simulink library "Pathfinding_lib"  (R2023b)
settings: Solver=VariableStepAuto  StartTime=0.0  StopTime=10.0  RelTol=1e-3
undefined symbols (not defined in the file): Spline_Max_Num_RefPoses, Spline_Num_Samples, Spline_Samples_Per_Pass, Spline_Tension, Spline_Velocity_Adjustment_Magnitude
libraries: $bdroot x39, simulink x4, matrix_library x1
settings Model: Creator=FIRSTMentor  LastModifiedBy=FIRSTMentor

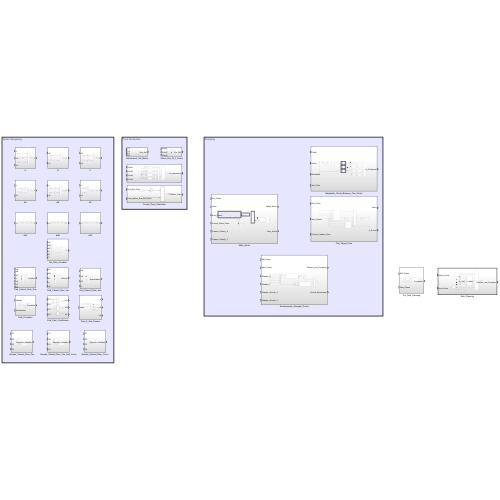
[thumbnail: Simulink's stored preview of the top-level diagram]
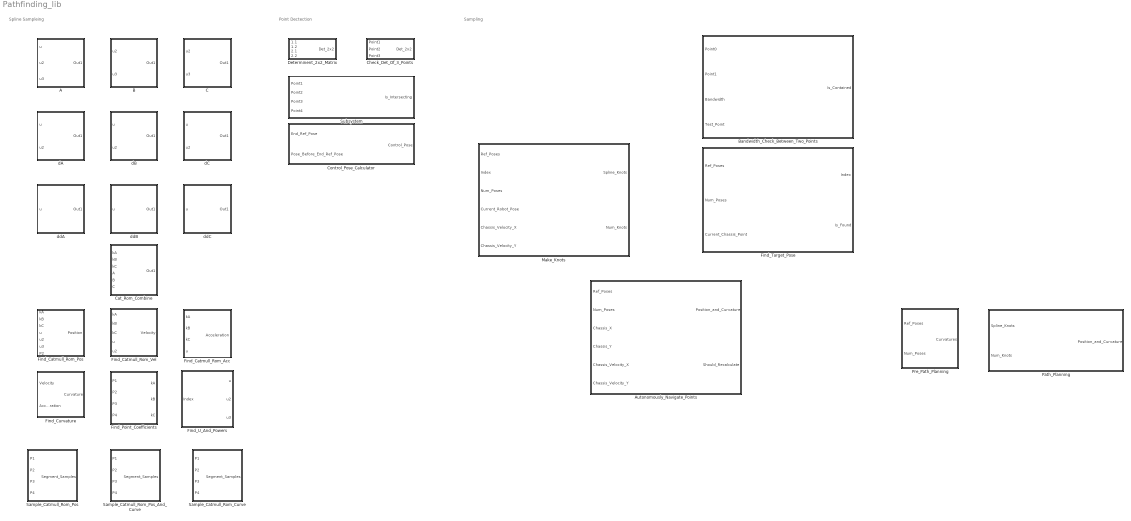
== system Pathfinding_lib ==
  note: Sampling
  note: Point Dectection
  note: Spline Sampleing
  A : Subsystem
  Autonomously_Navigate_Points : Subsystem
  B : Subsystem
  Bandwidth_Check_Between_Two_Points : Subsystem
  C : Subsystem
  Cat_Rom_Combine : Subsystem
  Check_Det_Of_3_Points : Subsystem
  Control_Pose_Calculator : Subsystem
  Determinent_2x2_Matrix : Subsystem
  Find_Catmull_Rom_Acc : Subsystem
  Find_Catmull_Rom_Pos : Subsystem
  Find_Catmull_Rom_Vel : Subsystem
  Find_Curvature : Subsystem
  Find_Point_Coefficients : Subsystem
  Find_Target_Pose : Subsystem
  Find_U_And_Powers : Subsystem
  Make_Knots : Subsystem
  Path_Planning : Subsystem  TreatAsAtomicUnit=on
  Pre_Path_Planning : Subsystem
  Sample_Catmull_Rom_Curve : Subsystem
  Sample_Catmull_Rom_Pos : Subsystem
  Sample_Catmull_Rom_Pos_And_Curve : Subsystem
  Subsystem : Subsystem
  dA : Subsystem
  dB : Subsystem
  dC : Subsystem
  ddA : Subsystem
  ddB : Subsystem
  ddC : Subsystem

== system Pathfinding_lib/A ==
  u : Inport
  u2 : Inport  Port=2
  u3 : Inport  Port=3
  Add : Sum  Inputs=+-+
  Gain : Gain  Gain=2
  Out1 : Outport
  wires:
  Add/1 -> Out1/1
  u/1 -> Add/1
  u2/1 -> Gain/1
  Gain/1 -> Add/2
  u3/1 -> Add/3

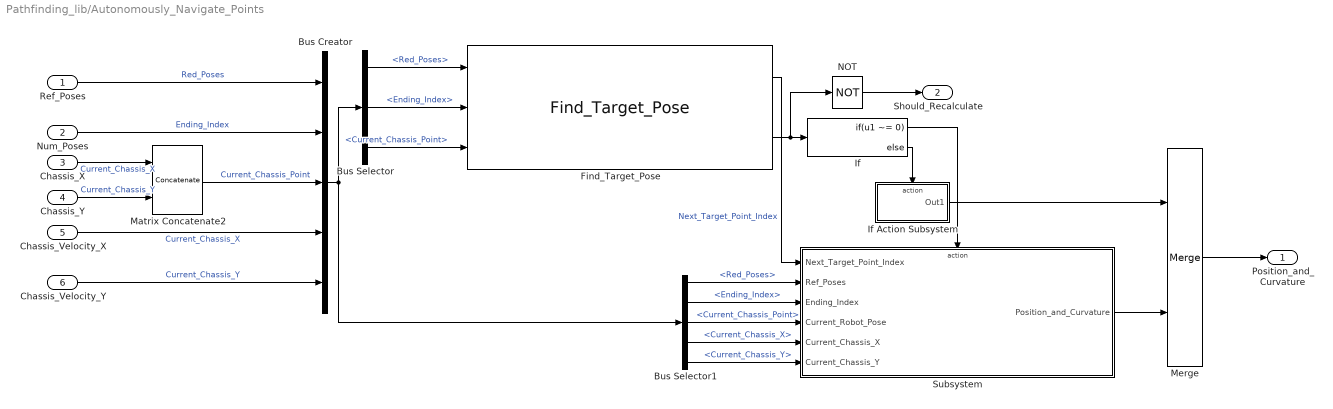
== system Pathfinding_lib/Autonomously_Navigate_Points ==
  Ref_Poses : Inport  OutDataTypeStr=double  PortDimensions=[Spline_Max_Num_RefPoses 2]
  Num_Poses : Inport  Port=2  OutDataTypeStr=int32  Unit=1  PortDimensions=1
  Chassis_X : Inport  Port=3  OutDataTypeStr=double  Unit=m  PortDimensions=1
  Chassis_Y : Inport  Port=4  OutDataTypeStr=double  Unit=m  PortDimensions=1
  Chassis_Velocity_X : Inport  Port=5  OutDataTypeStr=double  Unit=m  PortDimensions=1
  Chassis_Velocity_Y : Inport  Port=6  OutDataTypeStr=double  Unit=m  PortDimensions=1
  Bus Creator : BusCreator  Inputs=5
  Bus Selector : BusSelector  OutputSignals=Red_Poses,Ending_Index,Current_Chassis_Point
  Bus Selector1 : BusSelector  OutputSignals=Red_Poses,Ending_Index,Current_Chassis_Point,Current_Chassis_X,Current_Chassis_Y
  Find_Target_Pose : $bdroot/Find_Target_Pose  SystemSampleTime=-1  VariantActivationTime=update diagram  AllowFlexibleInterface=on  Latency=0  AutoFrameSizeCalculation=off
  If : If  IfExpression=u1 ~= 0
  If Action Subsystem : Subsystem  TreatAsAtomicUnit=on
  Matrix Concatenate2 : Concatenate  Mode=Multidimensional array  ConcatenateDimension=2
  Merge : Merge
  NOT : Logic  Operator=NOT  IconShape=distinctive  AllPortsSameDT=off  OutDataTypeStr=boolean
  Subsystem : Subsystem
  Position_and_Curvature : Outport  PortDimensions=[Spline_Num_Samples,3,2]
  Should_Recalculate : Outport  Port=2
  wires:
  Chassis_X/1 -> Matrix Concatenate2/1  "Current_Chassis_X"
  Chassis_Y/1 -> Matrix Concatenate2/2  "Current_Chassis_Y"
  Ref_Poses/1 -> Bus Creator/1  "Red_Poses"
  Matrix Concatenate2/1 -> Bus Creator/3  "Current_Chassis_Point"
  Num_Poses/1 -> Bus Creator/2  "Ending_Index"
  Find_Target_Pose/2 -> NOT/1, If/1
  Find_Target_Pose/1 -> Subsystem/1(Next_Target_Point_Index)  "Next_Target_Point_Index"
  Chassis_Velocity_X/1 -> Bus Creator/4  "Current_Chassis_X"
  Chassis_Velocity_Y/1 -> Bus Creator/5  "Current_Chassis_Y"
  Subsystem/1(Position_and_Curvature) -> Merge/2
  If/1 -> Subsystem/Action
  Bus Creator/1 -> Bus Selector1/1, Bus Selector/1
  Bus Selector/1 -> Find_Target_Pose/1  "<Red_Poses>"
  Bus Selector/2 -> Find_Target_Pose/2  "<Ending_Index>"
  Bus Selector/3 -> Find_Target_Pose/3  "<Current_Chassis_Point>"
  Bus Selector1/1 -> Subsystem/2(Ref_Poses)  "<Red_Poses>"
  Bus Selector1/2 -> Subsystem/3(Ending_Index)  "<Ending_Index>"
  Bus Selector1/3 -> Subsystem/4(Current_Robot_Pose)  "<Current_Chassis_Point>"
  Bus Selector1/4 -> Subsystem/5(Current_Chassis_X)  "<Current_Chassis_X>"
  Bus Selector1/5 -> Subsystem/6(Current_Chassis_Y)  "<Current_Chassis_Y>"
  NOT/1 -> Should_Recalculate/1
  If/2 -> If Action Subsystem/Action
  If Action Subsystem/1(Out1) -> Merge/1
  Merge/1 -> Position_and_Curvature/1

== system Pathfinding_lib/B ==
  u2 : Inport
  u3 : Inport  Port=2
  Add : Sum  Inputs=+-
  Out1 : Outport
  wires:
  Add/1 -> Out1/1
  u3/1 -> Add/2
  u2/1 -> Add/1

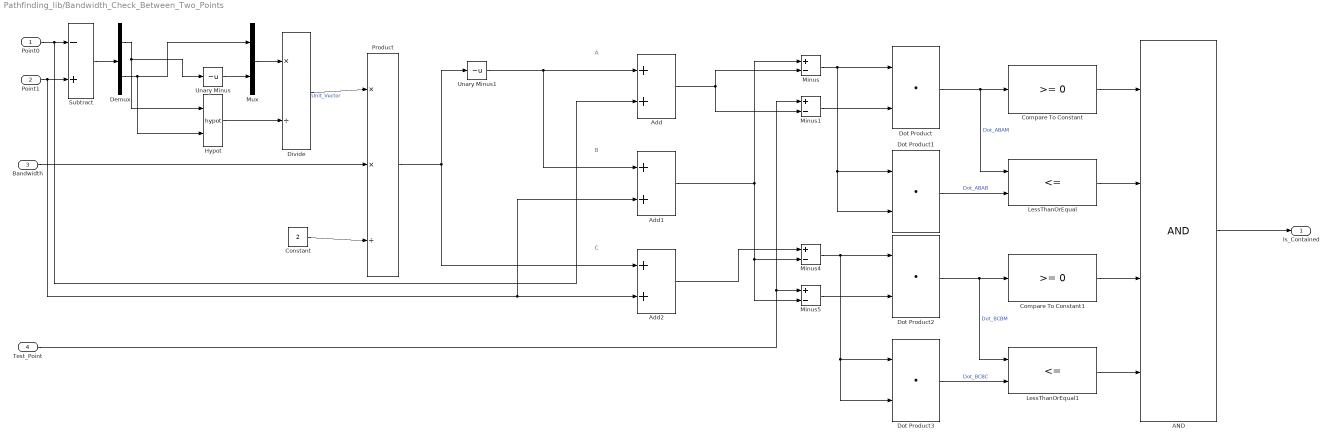
== system Pathfinding_lib/Bandwidth_Check_Between_Two_Points ==
  note: A
  note: B
  note: C
  Point0 : Inport  Unit=m  PortDimensions=[1 2]
  Point1 : Inport  Port=2  Unit=m  PortDimensions=[1 2]
  Bandwidth : Inport  Port=3  PortDimensions=1
  Test_Point : Inport  Port=4  Unit=m  PortDimensions=[1 2]
  AND : Logic  Inputs=4  IconShape=distinctive  AllPortsSameDT=off  OutDataTypeStr=boolean
  Add : Sum
  Add1 : Sum
  Add2 : Sum
  Compare To Constant : simulink/Logic and Bit Operations/Compare To Constant  relop=>=  const=0  OutDataTypeStr=boolean
  Compare To Constant1 : simulink/Logic and Bit Operations/Compare To Constant  relop=>=  const=0  OutDataTypeStr=boolean
  Constant : Constant  Value=2
  Demux : Demux  Outputs=2
  Divide : Product  Inputs=*/
  Dot Product{,1..3} (4 alike) : DotProduct  OutDataTypeStr=Inherit: Inherit via internal rule
  Hypot : Math  Operator=hypot
  LessThanOrEqual : RelationalOperator  Operator=<=  OutDataTypeStr=boolean  RndMeth=Simplest  InputSameDT=off
  LessThanOrEqual1 : RelationalOperator  Operator=<=  OutDataTypeStr=boolean  RndMeth=Simplest  InputSameDT=off
  Minus{,1,4..5} (4 alike) : Sum  Inputs=+-
  Mux : Mux  Inputs=2
  Product : Product  Inputs=**/
  Subtract : Sum  Inputs=-+
  Unary Minus : UnaryMinus
  Unary Minus1 : UnaryMinus
  Is_Contained : Outport
  wires:
  Point0/1 -> Add/2, Subtract/1
  Point1/1 -> Subtract/2, Add1/2, Add2/2
  Subtract/1 -> Demux/1
  Demux/2 -> Hypot/2, Mux/1
  Unary Minus/1 -> Mux/2
  Demux/1 -> Hypot/1, Unary Minus/1
  Mux/1 -> Divide/1
  Hypot/1 -> Divide/2
  Divide/1 -> Product/1  "Unit_Vector"
  Bandwidth/1 -> Product/2
  Constant/1 -> Product/3
  Product/1 -> Add2/1, Unary Minus1/1
  Unary Minus1/1 -> Add1/1, Add/1
  Minus1/1 -> Dot Product/2
  Dot Product/1 -> LessThanOrEqual/1, Compare To Constant/1  "Dot_ABAM"
  Dot Product1/1 -> LessThanOrEqual/2  "Dot_ABAB"
  Minus/1 -> Dot Product1/2, Dot Product1/1, Dot Product/1
  Dot Product2/1 -> Compare To Constant1/1, LessThanOrEqual1/1  "Dot_BCBM"
  Minus5/1 -> Dot Product2/2
  Dot Product3/1 -> LessThanOrEqual1/2  "Dot_BCBC"
  Minus4/1 -> Dot Product3/1, Dot Product3/2, Dot Product2/1
  Add1/1 -> Minus5/2, Minus4/2, Minus/1
  Add/1 -> Minus1/2, Minus/2
  Add2/1 -> Minus4/1
  Test_Point/1 -> Minus1/1, Minus5/1
  AND/1 -> Is_Contained/1
  Compare To Constant/1 -> AND/1
  Compare To Constant1/1 -> AND/3
  LessThanOrEqual/1 -> AND/2
  LessThanOrEqual1/1 -> AND/4

== system Pathfinding_lib/C ==
  u2 : Inport
  u3 : Inport  Port=2
  Add : Sum  Inputs=+-
  Gain : Gain  Gain=3
  Gain1 : Gain  Gain=2
  Out1 : Outport
  wires:
  u2/1 -> Gain/1
  u3/1 -> Gain1/1
  Gain/1 -> Add/1
  Gain1/1 -> Add/2
  Add/1 -> Out1/1

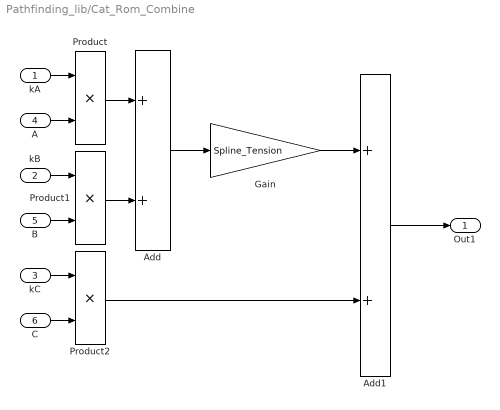
== system Pathfinding_lib/Cat_Rom_Combine ==
  kA : Inport
  kB : Inport  Port=2
  kC : Inport  Port=3
  A : Inport  Port=4
  B : Inport  Port=5
  C : Inport  Port=6
  Add : Sum  Inputs=2
  Add1 : Sum
  Gain : Gain  Gain=Spline_Tension
  Product : Product
  Product1 : Product
  Product2 : Product
  Out1 : Outport
  wires:
  kA/1 -> Product/1
  A/1 -> Product/2
  kC/1 -> Product2/1
  C/1 -> Product2/2
  kB/1 -> Product1/1
  B/1 -> Product1/2
  Product/1 -> Add/1
  Product1/1 -> Add/2
  Product2/1 -> Add1/2
  Add/1 -> Gain/1
  Add1/1 -> Out1/1
  Gain/1 -> Add1/1

== system Pathfinding_lib/Check_Det_Of_3_Points ==
  Point1 : Inport
  Point2 : Inport  Port=2
  Point3 : Inport  Port=3
  Demux : Demux  Outputs=2
  Demux1 : Demux  Outputs=2
  Demux2 : Demux  Outputs=2
  Determinent_2x2_Matrix : $bdroot/Determinent_2x2_Matrix  SystemSampleTime=-1  VariantActivationTime=update diagram  Latency=0  AutoFrameSizeCalculation=off
  Minus{,1..3} (4 alike) : Sum  Inputs=+-
  Det_2x2 : Outport
  wires:
  Determinent_2x2_Matrix/1 -> Det_2x2/1
  Minus/1 -> Determinent_2x2_Matrix/1
  Minus1/1 -> Determinent_2x2_Matrix/2
  Minus2/1 -> Determinent_2x2_Matrix/3
  Minus3/1 -> Determinent_2x2_Matrix/4
  Point1/1 -> Demux/1  "Point1"
  Point2/1 -> Demux1/1  "Point2"
  Point3/1 -> Demux2/1  "Point3"
  Demux/1 -> Minus/1  "Point1_X"
  Demux/2 -> Minus2/1  "Point1_Y"
  Demux1/1 -> Minus1/1  "Point2_X"
  Demux1/2 -> Minus3/1  "Point2_Y"
  Demux2/1 -> Minus2/2, Minus1/2, Minus/2  "Point3_X"
  Demux2/2 -> Minus3/2  "Point3_Y"

== system Pathfinding_lib/Control_Pose_Calculator ==
  End_Ref_Pose : Inport
  Pose_Before_End_Ref_Pose : Inport  Port=2
  Gain : Gain  Gain=2
  Subtract : Sum  Inputs=+-
  Control_Pose : Outport
  wires:
  End_Ref_Pose/1 -> Gain/1
  Gain/1 -> Subtract/1
  Pose_Before_End_Ref_Pose/1 -> Subtract/2
  Subtract/1 -> Control_Pose/1

== system Pathfinding_lib/Determinent_2x2_Matrix ==
  1.1 : Inport
  1.2 : Inport  Port=2
  2.1 : Inport  Port=3
  2.2 : Inport  Port=4
  Minus : Sum  Inputs=+-
  Product : Product
  Product1 : Product
  Det_2x2 : Outport
  wires:
  1.1/1 -> Product/1
  2.2/1 -> Product/2
  1.2/1 -> Product1/1
  2.1/1 -> Product1/2
  Product/1 -> Minus/1
  Product1/1 -> Minus/2
  Minus/1 -> Det_2x2/1

== system Pathfinding_lib/Find_Catmull_Rom_Acc ==
  kA : Inport  PortDimensions=[1 2]
  kB : Inport  Port=2  PortDimensions=[1 2]
  kC : Inport  Port=3  PortDimensions=[1 2]
  u : Inport  Port=4  PortDimensions=1
  Cat_Rom_Combine : $bdroot/Cat_Rom_Combine  SystemSampleTime=-1  VariantActivationTime=update diagram  AllowFlexibleInterface=on  Latency=0  AutoFrameSizeCalculation=off
  ddA : $bdroot/ddA  SystemSampleTime=-1  VariantActivationTime=update diagram  AllowFlexibleInterface=on  Latency=0  AutoFrameSizeCalculation=off
  ddB : $bdroot/ddB  SystemSampleTime=-1  VariantActivationTime=update diagram  AllowFlexibleInterface=on  Latency=0  AutoFrameSizeCalculation=off
  ddC : $bdroot/ddC  SystemSampleTime=-1  VariantActivationTime=update diagram  AllowFlexibleInterface=on  Latency=0  AutoFrameSizeCalculation=off
  Acceleration : Outport
  wires:
  kA/1 -> Cat_Rom_Combine/1
  kB/1 -> Cat_Rom_Combine/2
  kC/1 -> Cat_Rom_Combine/3
  ddA/1 -> Cat_Rom_Combine/4
  ddB/1 -> Cat_Rom_Combine/5
  ddC/1 -> Cat_Rom_Combine/6
  Cat_Rom_Combine/1 -> Acceleration/1
  u/1 -> ddA/1, ddC/1, ddB/1

== system Pathfinding_lib/Find_Catmull_Rom_Pos ==
  kA : Inport  PortDimensions=[1 2]
  kB : Inport  Port=2  PortDimensions=[1 2]
  kC : Inport  Port=3  PortDimensions=[1 2]
  u : Inport  Port=4  PortDimensions=1
  u2 : Inport  Port=5  PortDimensions=1
  u3 : Inport  Port=6  PortDimensions=1
  P2 : Inport  Port=7  PortDimensions=[1 2]
  A : $bdroot/A  SystemSampleTime=-1  VariantActivationTime=update diagram  AllowFlexibleInterface=on  Latency=0  AutoFrameSizeCalculation=off
  B : $bdroot/B  SystemSampleTime=-1  VariantActivationTime=update diagram  AllowFlexibleInterface=on  Latency=0  AutoFrameSizeCalculation=off
  C : $bdroot/C  SystemSampleTime=-1  VariantActivationTime=update diagram  AllowFlexibleInterface=on  Latency=0  AutoFrameSizeCalculation=off
  Cat_Rom_Combine : $bdroot/Cat_Rom_Combine  SystemSampleTime=-1  VariantActivationTime=update diagram  AllowFlexibleInterface=on  Latency=0  AutoFrameSizeCalculation=off
  Sum : Sum  Inputs=|++
  Position : Outport
  wires:
  u/1 -> A/1
  u2/1 -> C/1, B/1, A/2
  u3/1 -> C/2, B/2, A/3
  kA/1 -> Cat_Rom_Combine/1
  kB/1 -> Cat_Rom_Combine/2
  kC/1 -> Cat_Rom_Combine/3
  A/1 -> Cat_Rom_Combine/4
  B/1 -> Cat_Rom_Combine/5
  C/1 -> Cat_Rom_Combine/6
  P2/1 -> Sum/2
  Cat_Rom_Combine/1 -> Sum/1
  Sum/1 -> Position/1

== system Pathfinding_lib/Find_Catmull_Rom_Vel ==
  kA : Inport  PortDimensions=[1 2]
  kB : Inport  Port=2  PortDimensions=[1 2]
  kC : Inport  Port=3  PortDimensions=[1 2]
  u : Inport  Port=4  PortDimensions=1
  u2 : Inport  Port=5  PortDimensions=1
  Cat_Rom_Combine : $bdroot/Cat_Rom_Combine  SystemSampleTime=-1  VariantActivationTime=update diagram  AllowFlexibleInterface=on  Latency=0  AutoFrameSizeCalculation=off
  dA : $bdroot/dA  SystemSampleTime=-1  VariantActivationTime=update diagram  AllowFlexibleInterface=on  Latency=0  AutoFrameSizeCalculation=off
  dB : $bdroot/dB  SystemSampleTime=-1  VariantActivationTime=update diagram  AllowFlexibleInterface=on  Latency=0  AutoFrameSizeCalculation=off
  dC : $bdroot/dC  SystemSampleTime=-1  VariantActivationTime=update diagram  AllowFlexibleInterface=on  Latency=0  AutoFrameSizeCalculation=off
  Velocity : Outport
  wires:
  kA/1 -> Cat_Rom_Combine/1
  kB/1 -> Cat_Rom_Combine/2
  kC/1 -> Cat_Rom_Combine/3
  dA/1 -> Cat_Rom_Combine/4
  dB/1 -> Cat_Rom_Combine/5
  dC/1 -> Cat_Rom_Combine/6
  Cat_Rom_Combine/1 -> Velocity/1
  u/1 -> dC/1, dB/1, dA/1
  u2/1 -> dC/2, dB/2, dA/2

== system Pathfinding_lib/Find_Curvature ==
  Velocity : Inport  PortDimensions=[1 2]
  Acceleration : Inport  Port=2  PortDimensions=[1 2]
  Abs : Abs  SaturateOnIntegerOverflow=off
  Constant1 : Constant  Value=3
  Demux : Demux  Outputs=2
  Divide : Product  Inputs=*/
  Hypot : Math  Operator=hypot
  MATLAB Function : MATLAB Function  TreatAsAtomicUnit=on
  Matrix Concatenate : Concatenate  Mode=Multidimensional array
  Power1 : Math  Operator=pow
  Curvature : Outport  PortDimensions=1
  wires:
  Divide/1 -> Curvature/1
  Velocity/1 -> Demux/1, Matrix Concatenate/1
  Acceleration/1 -> Matrix Concatenate/2
  Matrix Concatenate/1 -> MATLAB Function/1(u)
  MATLAB Function/1(y) -> Abs/1
  Constant1/1 -> Power1/2
  Hypot/1 -> Power1/1
  Abs/1 -> Divide/1
  Power1/1 -> Divide/2
  Demux/1 -> Hypot/1
  Demux/2 -> Hypot/2

== system Pathfinding_lib/Find_Point_Coefficients ==
  P1 : Inport
  P2 : Inport  Port=2
  P3 : Inport  Port=3
  P4 : Inport  Port=4
  Minus : Sum  Inputs=+-
  Minus1 : Sum  Inputs=+-
  Minus2 : Sum  Inputs=+-
  kA : Outport
  kB : Outport  Port=2
  kC : Outport  Port=3
  wires:
  P2/1 -> Minus2/2, Minus1/1
  P1/1 -> Minus/2
  P3/1 -> Minus2/1, Minus/1
  P4/1 -> Minus1/2
  Minus/1 -> kA/1
  Minus1/1 -> kB/1
  Minus2/1 -> kC/1

== system Pathfinding_lib/Find_Target_Pose ==
  Ref_Poses : Inport  OutDataTypeStr=double  PortDimensions=[Spline_Max_Num_RefPoses 2]
  Num_Poses : Inport  Port=2  Unit=1  PortDimensions=1
  Current_Chassis_Point : Inport  Port=3  OutDataTypeStr=double  Unit=m  PortDimensions=[1 2]
  Bandwidth : Constant  Value=2
  Circle_Checks : Subsystem  TreatAsAtomicUnit=on
  Constant : Constant
  If : If  IfExpression=u1 == 0  ShowElse=off
  OR : Logic  Operator=OR  IconShape=distinctive  AllPortsSameDT=off  OutDataTypeStr=boolean
  Rectangle_Checks : Subsystem  TreatAsAtomicUnit=on
  Sum : Sum  Inputs=|++  OutDataTypeStr=int32
  Switch : Switch  Criteria=u2 ~= 0  SaturateOnIntegerOverflow=off  InputSameDT=off
  Index : Outport
  Is_Found : Outport  Port=2
  wires:
  Rectangle_Checks/2(Is_Found) -> Switch/2, OR/1, If/1
  Switch/1 -> Sum/1
  If/1 -> Circle_Checks/Action
  Num_Poses/1 -> Rectangle_Checks/2(Num_Poses), Circle_Checks/2(Num_Poses)  "Ending_Index"
  Current_Chassis_Point/1 -> Rectangle_Checks/3(Test_Point), Circle_Checks/3(Test_Point)  "Current_Chassis_Point"
  Ref_Poses/1 -> Rectangle_Checks/1(Ref_Poses), Circle_Checks/1(Ref_Poses)
  Rectangle_Checks/1(Index) -> Switch/1
  Circle_Checks/1(Index) -> Switch/3
  Bandwidth/1 -> Rectangle_Checks/4(Bandwidth), Circle_Checks/4(Bandwidth)
  Sum/1 -> Index/1  "Next_Target_Point_Index"
  OR/1 -> Is_Found/1
  Circle_Checks/2(Is_Found) -> OR/2
  Constant/1 -> Sum/2

== system Pathfinding_lib/Find_U_And_Powers ==
  Index : Inport
  Bias : Bias  Bias=-1  SaturateOnIntegerOverflow=off
  Constant : Constant  Value=2
  Constant1 : Constant  Value=3
  Constant2 : Constant  Value=Spline_Num_Samples-1
  Divide : Product  Inputs=*/
  Power : Math  Operator=pow
  Power1 : Math  Operator=pow
  u : Outport
  u2 : Outport  Port=2
  u3 : Outport  Port=3
  wires:
  Bias/1 -> Divide/1
  Constant2/1 -> Divide/2
  Power/1 -> u2/1  "u2"
  Power1/1 -> u3/1  "u3"
  Constant/1 -> Power/2
  Divide/1 -> u/1, Power1/1, Power/1  "u"
  Constant1/1 -> Power1/2
  Index/1 -> Bias/1

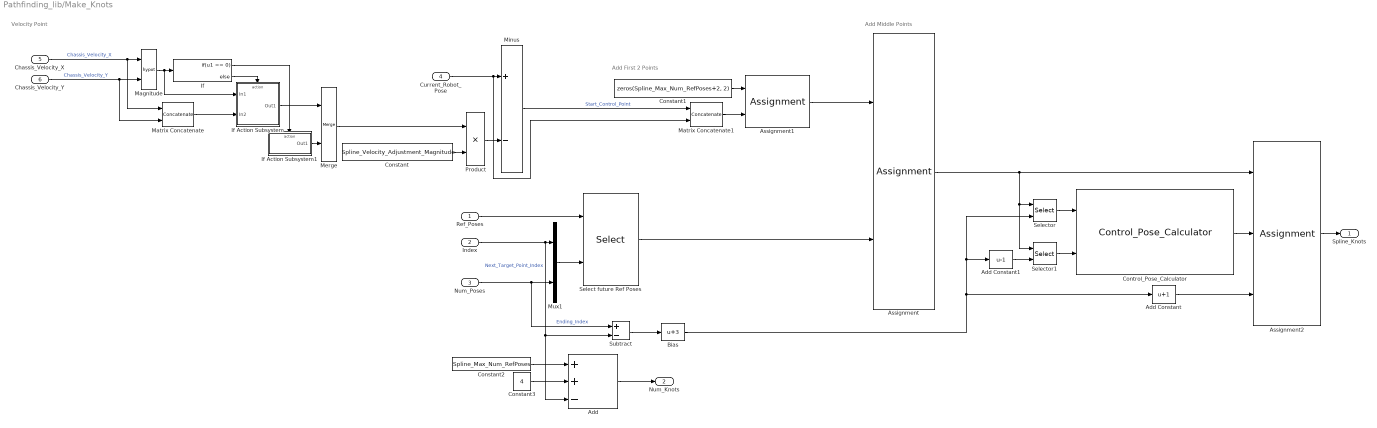
== system Pathfinding_lib/Make_Knots ==
  note: Add Middle Points
  note: Add First 2 Points
  note: Velocity Point
  Ref_Poses : Inport
  Index : Inport  Port=2
  Num_Poses : Inport  Port=3
  Current_Robot_Pose : Inport  Port=4
  Chassis_Velocity_X : Inport  Port=5
  Chassis_Velocity_Y : Inport  Port=6
  Add : Sum  Inputs=++-
  Add Constant : Bias  Bias=1  SaturateOnIntegerOverflow=off
  Add Constant1 : Bias  Bias=-1  SaturateOnIntegerOverflow=off
  Assignment : Assignment  NumberOfDimensions=2  DiagnosticForDimensions=Warning  IndexOptions=Starting index (dialog),Assign all  Indices=3,1  OutputSizes=1,1
  Assignment1 : Assignment  NumberOfDimensions=2  DiagnosticForDimensions=Warning  IndexOptions=Starting index (dialog),Assign all  Indices=1,1  OutputSizes=1,1
  Assignment2 : Assignment  NumberOfDimensions=2  DiagnosticForDimensions=Warning  IndexOptions=Index vector (port),Assign all  Indices=1,1  OutputSizes=1,1
  Bias : Bias  Bias=3  SaturateOnIntegerOverflow=off
  Constant : Constant  Value=Spline_Velocity_Adjustment_Magnitude
  Constant1 : Constant  Value=zeros(Spline_Max_Num_RefPoses+2, 2)
  Constant2 : Constant  Value=Spline_Max_Num_RefPoses
  Constant3 : Constant  Value=4
  Control_Pose_Calculator : $bdroot/Control_Pose_Calculator  SystemSampleTime=-1  VariantActivationTime=update diagram  AllowFlexibleInterface=on  Latency=0  AutoFrameSizeCalculation=off
  If : If  IfExpression=u1 == 0
  If Action Subsystem : Subsystem  TreatAsAtomicUnit=on
  If Action Subsystem1 : Subsystem  TreatAsAtomicUnit=on
  Magnitude : Math  Operator=hypot
  Matrix Concatenate : Concatenate  Mode=Multidimensional array  ConcatenateDimension=2
  Matrix Concatenate1 : Concatenate  Mode=Multidimensional array
  Merge : Merge
  Minus : Sum  Inputs=+-
  Mux1 : Mux  Inputs=2
  Product : Product
  Select future Ref Poses : Selector  NumberOfDimensions=2  InputPortWidth=3  IndexOptions=Starting and ending indices (port),Select all  Indices=[1 3],1  OutputSizes=1,1
  Selector : Selector  NumberOfDimensions=2  InputPortWidth=3  IndexOptions=Index vector (port),Select all  Indices=[1 3],1  OutputSizes=1,1
  Selector1 : Selector  NumberOfDimensions=2  InputPortWidth=3  IndexOptions=Index vector (port),Select all  Indices=[1 3],1  OutputSizes=1,1
  Subtract : Sum  Inputs=+-
  Spline_Knots : Outport
  Num_Knots : Outport  Port=2
  wires:
  Minus/1 -> Matrix Concatenate1/1  "Start_Control_Point"
  Matrix Concatenate1/1 -> Assignment1/2
  Selector/1 -> Control_Pose_Calculator/1
  Add Constant/1 -> Assignment2/3
  Product/1 -> Minus/2
  Current_Robot_Pose/1 -> Matrix Concatenate1/2, Minus/1
  Assignment/1 -> Assignment2/1, Selector/1, Selector1/1
  Index/1 -> Subtract/2, Add/3, Mux1/1  "Next_Target_Point_Index"
  Matrix Concatenate/1 -> If Action Subsystem/2(In2)
  Selector1/1 -> Control_Pose_Calculator/2
  Magnitude/1 -> If Action Subsystem/1(In1), If/1
  Assignment1/1 -> Assignment/1
  Select future Ref Poses/1 -> Assignment/2
  Constant1/1 -> Assignment1/1
  Control_Pose_Calculator/1 -> Assignment2/2
  Chassis_Velocity_X/1 -> Matrix Concatenate/1, Magnitude/1  "Chassis_Velocity_X"
  Chassis_Velocity_Y/1 -> Matrix Concatenate/2, Magnitude/2  "Chassis_Velocity_Y"
  Mux1/1 -> Select future Ref Poses/2
  Constant/1 -> Product/2
  Num_Poses/1 -> Subtract/1, Mux1/2  "Ending_Index"
  Ref_Poses/1 -> Select future Ref Poses/1
  Assignment2/1 -> Spline_Knots/1
  Constant2/1 -> Add/1
  Constant3/1 -> Add/2
  Add/1 -> Num_Knots/1
  Bias/1 -> Selector/2, Add Constant1/1, Add Constant/1
  If/1 -> If Action Subsystem1/Action
  If/2 -> If Action Subsystem/Action
  If Action Subsystem/1(Out1) -> Merge/1
  If Action Subsystem1/1(Out1) -> Merge/2
  Merge/1 -> Product/1
  Subtract/1 -> Bias/1
  Add Constant1/1 -> Selector1/2

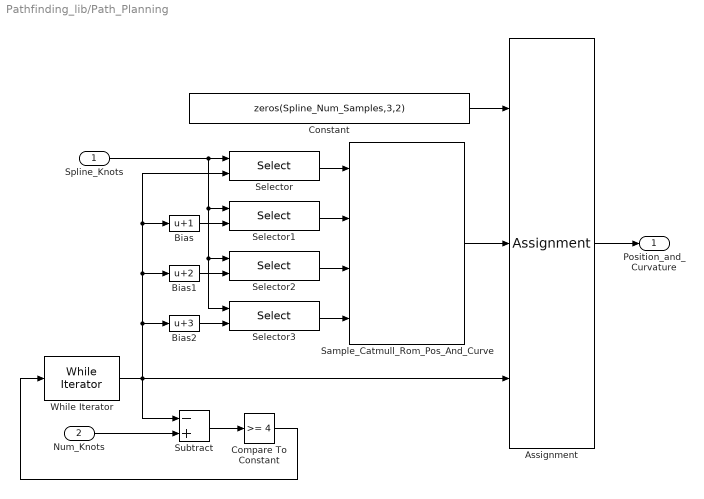
== system Pathfinding_lib/Path_Planning ==
  Spline_Knots : Inport
  Num_Knots : Inport  Port=2
  Assignment : Assignment  NumberOfDimensions=3  DiagnosticForDimensions=Warning  IndexOptions=Assign all,Assign all,Index vector (port)  Indices=1,1,1  OutputSizes=1,1,1
  Bias : Bias  Bias=1  SaturateOnIntegerOverflow=off
  Bias1 : Bias  Bias=2  SaturateOnIntegerOverflow=off
  Bias2 : Bias  Bias=3  SaturateOnIntegerOverflow=off
  Compare To Constant : simulink/Logic and Bit Operations/Compare To Constant  relop=>=  const=4  OutDataTypeStr=boolean
  Constant : Constant  Value=zeros(Spline_Num_Samples,3,2)  VectorParams1D=off
  Sample_Catmull_Rom_Pos_And_Curve : $bdroot/Sample_Catmull_Rom_Pos_And_Curve  SystemSampleTime=-1  VariantActivationTime=update diagram  AllowFlexibleInterface=on  Latency=0  AutoFrameSizeCalculation=off
  Selector{,1..3} (4 alike) : Selector  NumberOfDimensions=2  InputPortWidth=3  IndexOptions=Index vector (port),Select all  Indices=[1 3],1  OutputSizes=1,1
  Subtract : Sum  Inputs=-+
  While Iterator : WhileIterator  MaxIters=2  WhileBlockType=do-while  ShowIterationPort=on
  Position_and_Curvature : Outport
  wires:
  While Iterator/1 -> Subtract/1, Assignment/3, Bias2/1, Bias1/1, Bias/1, Selector/2
  Spline_Knots/1 -> Selector3/1, Selector2/1, Selector1/1, Selector/1
  Selector/1 -> Sample_Catmull_Rom_Pos_And_Curve/1
  Selector3/1 -> Sample_Catmull_Rom_Pos_And_Curve/4
  Selector2/1 -> Sample_Catmull_Rom_Pos_And_Curve/3
  Selector1/1 -> Sample_Catmull_Rom_Pos_And_Curve/2
  Bias2/1 -> Selector3/2
  Bias1/1 -> Selector2/2
  Bias/1 -> Selector1/2
  Sample_Catmull_Rom_Pos_And_Curve/1 -> Assignment/2
  Assignment/1 -> Position_and_Curvature/1
  Constant/1 -> Assignment/1
  Num_Knots/1 -> Subtract/2
  Subtract/1 -> Compare To Constant/1
  Compare To Constant/1 -> While Iterator/1

== system Pathfinding_lib/Pre_Path_Planning ==
  note: Num_Poses is Equal to Num_Knots in this case
  Ref_Poses : Inport  PortDimensions=[Spline_Samples_Per_Pass 3]
  Num_Poses : Inport  Port=2
  Find_Curvatures : Subsystem  TreatAsAtomicUnit=on
  Ref_Poses_To_Knots : Subsystem
  Curvatures : Outport
  wires:
  Ref_Poses/1 -> Ref_Poses_To_Knots/1(Ref_Poses)
  Ref_Poses_To_Knots/1(Knots) -> Find_Curvatures/1(Knots)
  Num_Poses/1 -> Find_Curvatures/2(Num_Knots), Ref_Poses_To_Knots/2(Num_Poses)
  Find_Curvatures/1(Curvatures) -> Curvatures/1

== system Pathfinding_lib/Sample_Catmull_Rom_Curve ==
  P1 : Inport  PortDimensions=[1 2]
  P2 : Inport  Port=2  PortDimensions=[1 2]
  P3 : Inport  Port=3  PortDimensions=[1 2]
  P4 : Inport  Port=4  PortDimensions=[1 2]
  Find_Point_Coefficients : $bdroot/Find_Point_Coefficients  SystemSampleTime=-1  VariantActivationTime=update diagram  AllowFlexibleInterface=on  Latency=0  AutoFrameSizeCalculation=off
  For Iterator Subsystem : Subsystem  TreatAsAtomicUnit=on
  Segment_Samples : Outport
  wires:
  P4/1 -> Find_Point_Coefficients/4  "P4"
  P3/1 -> Find_Point_Coefficients/3  "P3"
  P1/1 -> Find_Point_Coefficients/1  "P1"
  For Iterator Subsystem/1(Segment_Samples) -> Segment_Samples/1
  Find_Point_Coefficients/3 -> For Iterator Subsystem/3(kC)
  Find_Point_Coefficients/2 -> For Iterator Subsystem/2(kB)
  Find_Point_Coefficients/1 -> For Iterator Subsystem/1(kA)
  P2/1 -> Find_Point_Coefficients/2  "P2"

== system Pathfinding_lib/Sample_Catmull_Rom_Pos ==
  P1 : Inport  PortDimensions=[1 2]
  P2 : Inport  Port=2  PortDimensions=[1 2]
  P3 : Inport  Port=3  PortDimensions=[1 2]
  P4 : Inport  Port=4  PortDimensions=[1 2]
  Find_Point_Coefficients : $bdroot/Find_Point_Coefficients  SystemSampleTime=-1  VariantActivationTime=update diagram  AllowFlexibleInterface=on  Latency=0  AutoFrameSizeCalculation=off
  For Iterator Subsystem : Subsystem  TreatAsAtomicUnit=on
  Segment_Samples : Outport
  wires:
  P2/1 -> For Iterator Subsystem/4(P2), Find_Point_Coefficients/2  "P2"
  Find_Point_Coefficients/1 -> For Iterator Subsystem/1(kA)
  Find_Point_Coefficients/2 -> For Iterator Subsystem/2(kB)
  Find_Point_Coefficients/3 -> For Iterator Subsystem/3(kC)
  For Iterator Subsystem/1(Segment_Samples) -> Segment_Samples/1
  P1/1 -> Find_Point_Coefficients/1  "P1"
  P3/1 -> Find_Point_Coefficients/3  "P3"
  P4/1 -> Find_Point_Coefficients/4  "P4"

== system Pathfinding_lib/Sample_Catmull_Rom_Pos_And_Curve ==
  P1 : Inport  PortDimensions=[1 2]
  P2 : Inport  Port=2  PortDimensions=[1 2]
  P3 : Inport  Port=3  PortDimensions=[1 2]
  P4 : Inport  Port=4  PortDimensions=[1 2]
  Find_Point_Coefficients : $bdroot/Find_Point_Coefficients  SystemSampleTime=-1  VariantActivationTime=update diagram  AllowFlexibleInterface=on  Latency=0  AutoFrameSizeCalculation=off
  For Iterator Subsystem : Subsystem  TreatAsAtomicUnit=on
  Segment_Samples : Outport
  wires:
  P4/1 -> Find_Point_Coefficients/4  "P4"
  P3/1 -> Find_Point_Coefficients/3  "P3"
  P1/1 -> Find_Point_Coefficients/1  "P1"
  For Iterator Subsystem/1(Segment_Samples) -> Segment_Samples/1
  Find_Point_Coefficients/3 -> For Iterator Subsystem/3(kC)
  Find_Point_Coefficients/2 -> For Iterator Subsystem/2(kB)
  Find_Point_Coefficients/1 -> For Iterator Subsystem/1(kA)
  P2/1 -> Find_Point_Coefficients/2, For Iterator Subsystem/4(P2)  "P2"

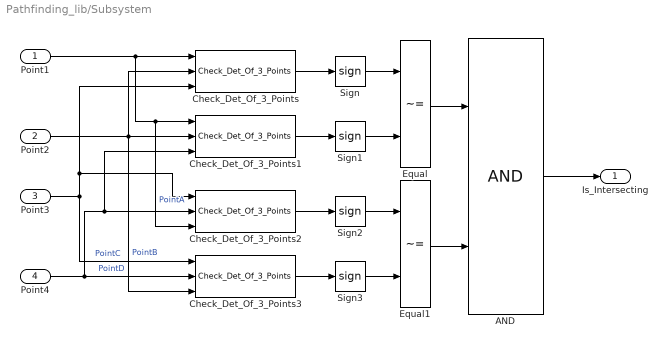
== system Pathfinding_lib/Subsystem ==
  Point1 : Inport  PortDimensions=2
  Point2 : Inport  Port=2  PortDimensions=2
  Point3 : Inport  Port=3  PortDimensions=2
  Point4 : Inport  Port=4  PortDimensions=2
  AND : Logic  IconShape=distinctive  AllPortsSameDT=off  OutDataTypeStr=boolean
  Check_Det_Of_3_Points{,1..3} (4 alike) : $bdroot/Check_Det_Of_3_Points  SystemSampleTime=-1  VariantActivationTime=update diagram  Latency=0  AutoFrameSizeCalculation=off
  Equal : RelationalOperator  Operator=~=  OutDataTypeStr=boolean  RndMeth=Simplest  InputSameDT=off
  Equal1 : RelationalOperator  Operator=~=  OutDataTypeStr=boolean  RndMeth=Simplest  InputSameDT=off
  Sign{,1..3} (4 alike) : Signum
  Is_Intersecting : Outport
  wires:
  Point1/1 -> Check_Det_Of_3_Points/1, Check_Det_Of_3_Points2/3, Check_Det_Of_3_Points1/1  "PointA"
  Point2/1 -> Check_Det_Of_3_Points/2, Check_Det_Of_3_Points1/2, Check_Det_Of_3_Points3/3  "PointB"
  Point3/1 -> Check_Det_Of_3_Points2/1, Check_Det_Of_3_Points/3, Check_Det_Of_3_Points3/1  "PointC"
  Point4/1 -> Check_Det_Of_3_Points3/2, Check_Det_Of_3_Points2/2, Check_Det_Of_3_Points1/3  "PointD"
  Check_Det_Of_3_Points/1 -> Sign/1
  Check_Det_Of_3_Points1/1 -> Sign1/1
  Check_Det_Of_3_Points2/1 -> Sign2/1
  Check_Det_Of_3_Points3/1 -> Sign3/1
  Sign/1 -> Equal/1
  Sign1/1 -> Equal/2
  Sign2/1 -> Equal1/1
  Sign3/1 -> Equal1/2
  Equal/1 -> AND/1
  Equal1/1 -> AND/2
  AND/1 -> Is_Intersecting/1

== system Pathfinding_lib/dA ==
  u : Inport
  u2 : Inport  Port=2
  Add : Sum  Inputs=-+
  Bias : Bias  Bias=1  SaturateOnIntegerOverflow=off
  Gain : Gain  Gain=4
  Gain1 : Gain  Gain=3
  Out1 : Outport
  wires:
  u2/1 -> Gain1/1
  u/1 -> Gain/1
  Bias/1 -> Out1/1
  Gain/1 -> Add/1
  Add/1 -> Bias/1
  Gain1/1 -> Add/2

== system Pathfinding_lib/dB ==
  u : Inport
  u2 : Inport  Port=2
  Add : Sum  Inputs=+-
  Gain : Gain  Gain=2
  Gain1 : Gain  Gain=3
  Out1 : Outport
  wires:
  u2/1 -> Gain1/1
  u/1 -> Gain/1
  Gain/1 -> Add/1
  Gain1/1 -> Add/2
  Add/1 -> Out1/1

== system Pathfinding_lib/dC ==
  u : Inport
  u2 : Inport  Port=2
  Add : Sum  Inputs=+-
  Gain : Gain  Gain=6
  Out1 : Outport
  wires:
  Gain/1 -> Out1/1
  u/1 -> Add/1
  u2/1 -> Add/2
  Add/1 -> Gain/1

== system Pathfinding_lib/ddA ==
  u : Inport
  Bias : Bias  Bias=-4  SaturateOnIntegerOverflow=off
  Gain : Gain  Gain=6
  Out1 : Outport
  wires:
  Bias/1 -> Out1/1
  u/1 -> Gain/1
  Gain/1 -> Bias/1

== system Pathfinding_lib/ddB ==
  u : Inport
  Bias : Bias  Bias=2  SaturateOnIntegerOverflow=off
  Gain : Gain  Gain=-6
  Out1 : Outport
  wires:
  u/1 -> Gain/1
  Gain/1 -> Bias/1
  Bias/1 -> Out1/1

== system Pathfinding_lib/ddC ==
  u : Inport
  Bias : Bias  Bias=6  SaturateOnIntegerOverflow=off
  Gain : Gain  Gain=-12
  Out1 : Outport
  wires:
  u/1 -> Gain/1
  Gain/1 -> Bias/1
  Bias/1 -> Out1/1

== system Pathfinding_lib/Autonomously_Navigate_Points/If Action Subsystem ==
  Action Port : ActionPort  ActionPortLabel=else
  Constant : Constant  Value=zeros(Spline_Num_Samples,3,2)
  Out1 : Outport
  wires:
  Constant/1 -> Out1/1

== system Pathfinding_lib/Autonomously_Navigate_Points/Subsystem ==
  Next_Target_Point_Index : Inport
  Ref_Poses : Inport  Port=2
  Ending_Index : Inport  Port=3
  Current_Robot_Pose : Inport  Port=4
  Current_Chassis_X : Inport  Port=5
  Current_Chassis_Y : Inport  Port=6
  Action Port : ActionPort  PropagateVarSize=During execution  ActionPortLabel=if(u1 ~= 0)
  Make_Knots : $bdroot/Make_Knots  SystemSampleTime=-1  VariantActivationTime=update diagram  AllowFlexibleInterface=on  Latency=0  AutoFrameSizeCalculation=off
  Path_Planning : $bdroot/Path_Planning  SystemSampleTime=-1  VariantActivationTime=update diagram  AllowFlexibleInterface=on  Latency=0  AutoFrameSizeCalculation=off
  Position_and_Curvature : Outport  PortDimensions=[Spline_Num_Samples,3,2]
  wires:
  Current_Chassis_Y/1 -> Make_Knots/6
  Current_Robot_Pose/1 -> Make_Knots/4
  Ref_Poses/1 -> Make_Knots/1
  Current_Chassis_X/1 -> Make_Knots/5
  Next_Target_Point_Index/1 -> Make_Knots/2
  Ending_Index/1 -> Make_Knots/3
  Make_Knots/1 -> Path_Planning/1
  Make_Knots/2 -> Path_Planning/2
  Path_Planning/1 -> Position_and_Curvature/1

== system Pathfinding_lib/Find_Target_Pose/Circle_Checks ==
  Ref_Poses : Inport
  Num_Poses : Inport  Port=2
  Test_Point : Inport  Port=3
  Bandwidth : Inport  Port=4
  Action Port : ActionPort  ActionPortLabel=if(u1 == 1)
  Circle_Checks : Subsystem  TreatAsAtomicUnit=on
  Index : Outport
  Is_Found : Outport  Port=2
  wires:
  Ref_Poses/1 -> Circle_Checks/1(Ref_Poses)
  Test_Point/1 -> Circle_Checks/3(Test_Point)
  Bandwidth/1 -> Circle_Checks/4(Bandwidth)
  Circle_Checks/1(Index) -> Index/1
  Num_Poses/1 -> Circle_Checks/2(Num_Poses)
  Circle_Checks/2(Is_Found) -> Is_Found/1

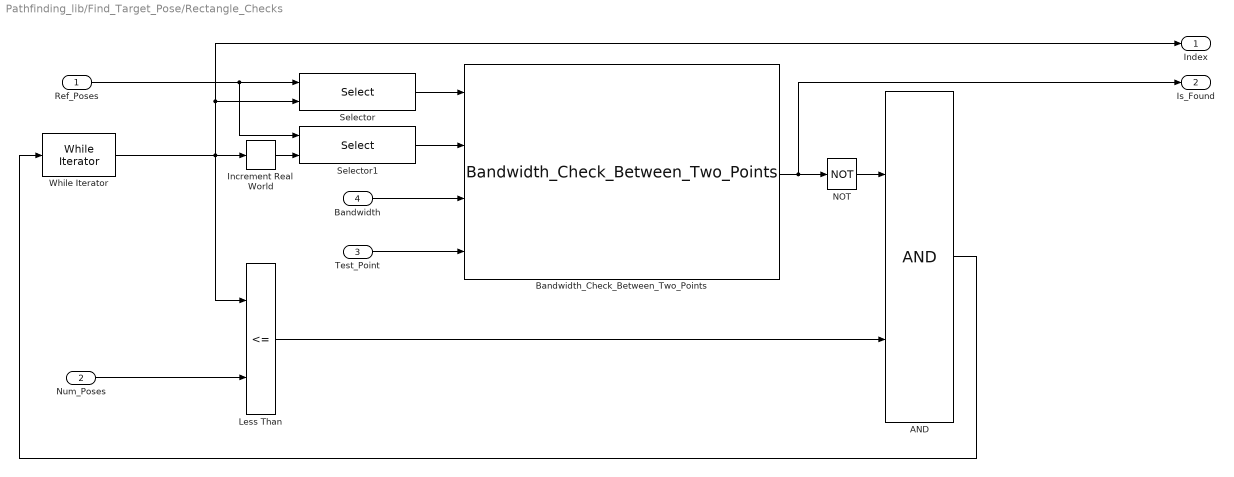
== system Pathfinding_lib/Find_Target_Pose/Rectangle_Checks ==
  Ref_Poses : Inport
  Num_Poses : Inport  Port=2
  Test_Point : Inport  Port=3
  Bandwidth : Inport  Port=4
  AND : Logic  IconShape=distinctive  AllPortsSameDT=off  OutDataTypeStr=boolean
  Bandwidth_Check_Between_Two_Points : $bdroot/Bandwidth_Check_Between_Two_Points  SystemSampleTime=-1  VariantActivationTime=update diagram  AllowFlexibleInterface=on  Latency=0  AutoFrameSizeCalculation=off
  Increment Real World : simulink/Additional Math & Discrete/Additional Math: Increment - Decrement/Increment Real World
  Less Than : RelationalOperator  Operator=<=  OutDataTypeStr=boolean  RndMeth=Simplest  InputSameDT=off
  NOT : Logic  Operator=NOT  IconShape=distinctive  AllPortsSameDT=off  OutDataTypeStr=boolean
  Selector : Selector  NumberOfDimensions=2  InputPortWidth=3  IndexOptions=Index vector (port),Select all  Indices=[1 3],1  OutputSizes=1,1
  Selector1 : Selector  NumberOfDimensions=2  InputPortWidth=3  IndexOptions=Index vector (port),Select all  Indices=[1 3],1  OutputSizes=1,1
  While Iterator : WhileIterator  MaxIters=Spline_Max_Num_RefPoses-1  WhileBlockType=do-while  ShowIterationPort=on
  Index : Outport
  Is_Found : Outport  Port=2
  wires:
  Test_Point/1 -> Bandwidth_Check_Between_Two_Points/4
  Bandwidth/1 -> Bandwidth_Check_Between_Two_Points/3
  Selector/1 -> Bandwidth_Check_Between_Two_Points/1
  Selector1/1 -> Bandwidth_Check_Between_Two_Points/2
  Ref_Poses/1 -> Selector1/1, Selector/1
  NOT/1 -> AND/1
  Increment Real World/1 -> Selector1/2
  While Iterator/1 -> Less Than/1, Increment Real World/1, Index/1, Selector/2
  Bandwidth_Check_Between_Two_Points/1 -> Is_Found/1, NOT/1
  Less Than/1 -> AND/2
  AND/1 -> While Iterator/1
  Num_Poses/1 -> Less Than/2

== system Pathfinding_lib/Make_Knots/If Action Subsystem ==
  In1 : Inport
  In2 : Inport  Port=2
  Action Port : ActionPort  ActionPortLabel=else
  Unit_Vector : Product  Inputs=/*
  Out1 : Outport
  wires:
  In1/1 -> Unit_Vector/1
  In2/1 -> Unit_Vector/2
  Unit_Vector/1 -> Out1/1

== system Pathfinding_lib/Make_Knots/If Action Subsystem1 ==
  Action Port : ActionPort  ActionPortLabel=if(u1 > 0)
  Constant : Constant  Value=[0 0]  VectorParams1D=off
  Out1 : Outport
  wires:
  Constant/1 -> Out1/1

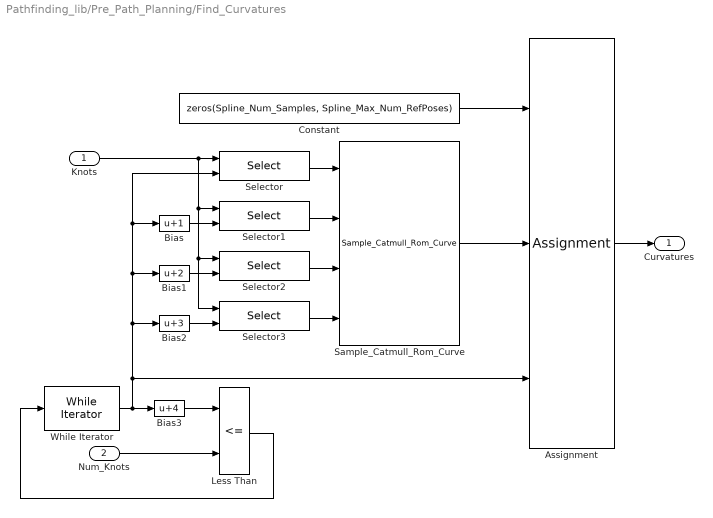
== system Pathfinding_lib/Pre_Path_Planning/Find_Curvatures ==
  Knots : Inport
  Num_Knots : Inport  Port=2
  Assignment : Assignment  NumberOfDimensions=2  DiagnosticForDimensions=Warning  IndexOptions=Assign all,Index vector (port)  Indices=1,1  OutputSizes=1,1
  Bias : Bias  Bias=1  SaturateOnIntegerOverflow=off
  Bias1 : Bias  Bias=2  SaturateOnIntegerOverflow=off
  Bias2 : Bias  Bias=3  SaturateOnIntegerOverflow=off
  Bias3 : Bias  Bias=4  SaturateOnIntegerOverflow=off
  Constant : Constant  Value=zeros(Spline_Num_Samples, Spline_Max_Num_RefPoses)  VectorParams1D=off
  Less Than : RelationalOperator  Operator=<=  OutDataTypeStr=boolean  RndMeth=Simplest  InputSameDT=off
  Sample_Catmull_Rom_Curve : $bdroot/Sample_Catmull_Rom_Curve  SystemSampleTime=-1  VariantActivationTime=update diagram  AllowFlexibleInterface=on  Latency=0  AutoFrameSizeCalculation=off
  Selector{,1..3} (4 alike) : Selector  NumberOfDimensions=2  InputPortWidth=3  IndexOptions=Index vector (port),Select all  Indices=[1 3],1  OutputSizes=1,1
  While Iterator : WhileIterator  MaxIters=-1  WhileBlockType=do-while  ShowIterationPort=on
  Curvatures : Outport
  wires:
  While Iterator/1 -> Bias3/1, Assignment/3, Bias2/1, Bias1/1, Bias/1, Selector/2
  Num_Knots/1 -> Less Than/2
  Less Than/1 -> While Iterator/1
  Knots/1 -> Selector3/1, Selector2/1, Selector1/1, Selector/1
  Selector/1 -> Sample_Catmull_Rom_Curve/1
  Selector3/1 -> Sample_Catmull_Rom_Curve/4
  Selector2/1 -> Sample_Catmull_Rom_Curve/3
  Selector1/1 -> Sample_Catmull_Rom_Curve/2
  Bias2/1 -> Selector3/2
  Bias1/1 -> Selector2/2
  Bias/1 -> Selector1/2
  Bias3/1 -> Less Than/1
  Sample_Catmull_Rom_Curve/1 -> Assignment/2
  Assignment/1 -> Curvatures/1
  Constant/1 -> Assignment/1

== system Pathfinding_lib/Pre_Path_Planning/Ref_Poses_To_Knots ==
  Ref_Poses : Inport  PortDimensions=[Spline_Samples_Per_Pass 3]
  Num_Poses : Inport  Port=2
  Add_Control_Knot_At_End : Assignment  NumberOfDimensions=2  DiagnosticForDimensions=Warning  IndexOptions=Index vector (port),Assign all  Indices=2,1  OutputSizes=1,1
  Assignment : Assignment  NumberOfDimensions=2  DiagnosticForDimensions=Warning  IndexOptions=Starting index (dialog),Assign all  Indices=1,1  OutputSizes=1,1
  Bias : Bias  Bias=-1  SaturateOnIntegerOverflow=off
  Bias1 : Bias  Bias=-2  SaturateOnIntegerOverflow=off
  Calc_Control_Knot : $bdroot/Control_Pose_Calculator  SystemSampleTime=-1  VariantActivationTime=update diagram  AllowFlexibleInterface=on  Latency=0  AutoFrameSizeCalculation=off
  Empty_Poses : Constant  Value=zeros(Spline_Samples_Per_Pass,2)
  Extract_Poses : matrix_library/Submatrix  RowSpan=Range of rows  RowStartMode=Index  RowStartIndex=2  RowEndMode=Last  RowEndIndex=1  ColSpan=Range of columns  ColStartMode=First  ColStartIndex=1  ColEndMode=Index  ColEndIndex=2
  Selector : Selector  NumberOfDimensions=2  InputPortWidth=3  IndexOptions=Index vector (port),Select all  Indices=[1 3],1  OutputSizes=1,1
  Selector1 : Selector  NumberOfDimensions=2  InputPortWidth=3  IndexOptions=Index vector (port),Select all  Indices=[1 3],1  OutputSizes=1,1
  Knots : Outport
  wires:
  Empty_Poses/1 -> Assignment/1
  Ref_Poses/1 -> Extract_Poses/1
  Extract_Poses/1 -> Assignment/2
  Add_Control_Knot_At_End/1 -> Knots/1
  Calc_Control_Knot/1 -> Add_Control_Knot_At_End/2
  Selector/1 -> Calc_Control_Knot/1
  Selector1/1 -> Calc_Control_Knot/2
  Assignment/1 -> Selector/1, Add_Control_Knot_At_End/1, Selector1/1
  Num_Poses/1 -> Bias1/1, Add_Control_Knot_At_End/3, Bias/1
  Bias/1 -> Selector/2
  Bias1/1 -> Selector1/2

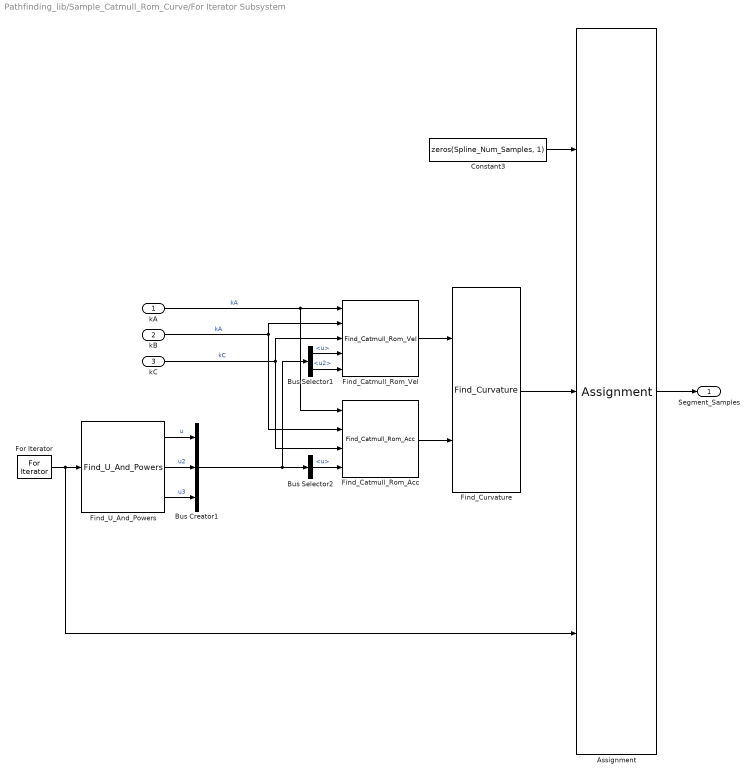
== system Pathfinding_lib/Sample_Catmull_Rom_Curve/For Iterator Subsystem ==
  kA : Inport  PortDimensions=[1 2]
  kB : Inport  Port=2  PortDimensions=[1 2]
  kC : Inport  Port=3  PortDimensions=[1 2]
  Assignment : Assignment  NumberOfDimensions=2  DiagnosticForDimensions=Warning  IndexOptions=Index vector (port),Assign all  Indices=1,1  OutputSizes=1,1
  Bus Creator1 : BusCreator  Inputs=3
  Bus Selector1 : BusSelector  OutputSignals=u,u2
  Bus Selector2 : BusSelector  OutputSignals=u
  Constant3 : Constant  Value=zeros(Spline_Num_Samples, 1)  VectorParams1D=off
  Find_Catmull_Rom_Acc : $bdroot/Find_Catmull_Rom_Acc  SystemSampleTime=-1  VariantActivationTime=update diagram  AllowFlexibleInterface=on  Latency=0  AutoFrameSizeCalculation=off
  Find_Catmull_Rom_Vel : $bdroot/Find_Catmull_Rom_Vel  SystemSampleTime=-1  VariantActivationTime=update diagram  AllowFlexibleInterface=on  Latency=0  AutoFrameSizeCalculation=off
  Find_Curvature : $bdroot/Find_Curvature  SystemSampleTime=-1  VariantActivationTime=update diagram  AllowFlexibleInterface=on  Latency=0  AutoFrameSizeCalculation=off
  Find_U_And_Powers : $bdroot/Find_U_And_Powers  SystemSampleTime=-1  VariantActivationTime=update diagram  AllowFlexibleInterface=on  Latency=0  AutoFrameSizeCalculation=off
  For Iterator : ForIterator  IterationLimit=Spline_Num_Samples
  Segment_Samples : Outport
  wires:
  Find_U_And_Powers/3 -> Bus Creator1/3  "u3"
  Find_U_And_Powers/1 -> Bus Creator1/1  "u"
  Find_U_And_Powers/2 -> Bus Creator1/2  "u2"
  Find_Curvature/1 -> Assignment/2
  Find_Catmull_Rom_Acc/1 -> Find_Curvature/2
  Find_Catmull_Rom_Vel/1 -> Find_Curvature/1
  kC/1 -> Find_Catmull_Rom_Vel/3, Find_Catmull_Rom_Acc/3  "kC"
  kB/1 -> Find_Catmull_Rom_Vel/2, Find_Catmull_Rom_Acc/2  "kA"
  kA/1 -> Find_Catmull_Rom_Vel/1, Find_Catmull_Rom_Acc/1  "kA"
  Bus Selector2/1 -> Find_Catmull_Rom_Acc/4  "<u>"
  Bus Selector1/2 -> Find_Catmull_Rom_Vel/5  "<u2>"
  Bus Selector1/1 -> Find_Catmull_Rom_Vel/4  "<u>"
  Bus Creator1/1 -> Bus Selector1/1, Bus Selector2/1
  Assignment/1 -> Segment_Samples/1
  Constant3/1 -> Assignment/1
  For Iterator/1 -> Assignment/3, Find_U_And_Powers/1
  ? -> ?

== system Pathfinding_lib/Sample_Catmull_Rom_Pos/For Iterator Subsystem ==
  kA : Inport  PortDimensions=[1 2]
  kB : Inport  Port=2  PortDimensions=[1 2]
  kC : Inport  Port=3  PortDimensions=[1 2]
  P2 : Inport  Port=4  PortDimensions=[1 2]
  Assignment : Assignment  NumberOfDimensions=2  DiagnosticForDimensions=Warning  IndexOptions=Index vector (port),Assign all  Indices=1,1  OutputSizes=1,1
  Bus Creator1 : BusCreator  Inputs=3
  Bus Selector : BusSelector  OutputSignals=u,u2,u3
  Constant3 : Constant  Value=zeros(Spline_Num_Samples, 2)
  Find_Catmull_Rom_Pos : $bdroot/Find_Catmull_Rom_Pos  SystemSampleTime=-1  VariantActivationTime=update diagram  AllowFlexibleInterface=on  Latency=0  AutoFrameSizeCalculation=off
  Find_U_And_Powers : $bdroot/Find_U_And_Powers  SystemSampleTime=-1  VariantActivationTime=update diagram  AllowFlexibleInterface=on  Latency=0  AutoFrameSizeCalculation=off
  For Iterator : ForIterator  IterationLimit=Spline_Num_Samples
  Segment_Samples : Outport
  wires:
  ? -> ?
  For Iterator/1 -> Find_U_And_Powers/1, Assignment/3
  Constant3/1 -> Assignment/1
  Assignment/1 -> Segment_Samples/1
  Bus Creator1/1 -> Bus Selector/1
  Bus Selector/1 -> Find_Catmull_Rom_Pos/4  "<u>"
  Bus Selector/3 -> Find_Catmull_Rom_Pos/6  "<u3>"
  Bus Selector/2 -> Find_Catmull_Rom_Pos/5  "<u2>"
  kA/1 -> Find_Catmull_Rom_Pos/1  "kA"
  kB/1 -> Find_Catmull_Rom_Pos/2  "kA"
  kC/1 -> Find_Catmull_Rom_Pos/3  "kC"
  Find_Catmull_Rom_Pos/1 -> Assignment/2
  P2/1 -> Find_Catmull_Rom_Pos/7  "kC"
  Find_U_And_Powers/2 -> Bus Creator1/2  "u2"
  Find_U_And_Powers/1 -> Bus Creator1/1  "u"
  Find_U_And_Powers/3 -> Bus Creator1/3  "u3"

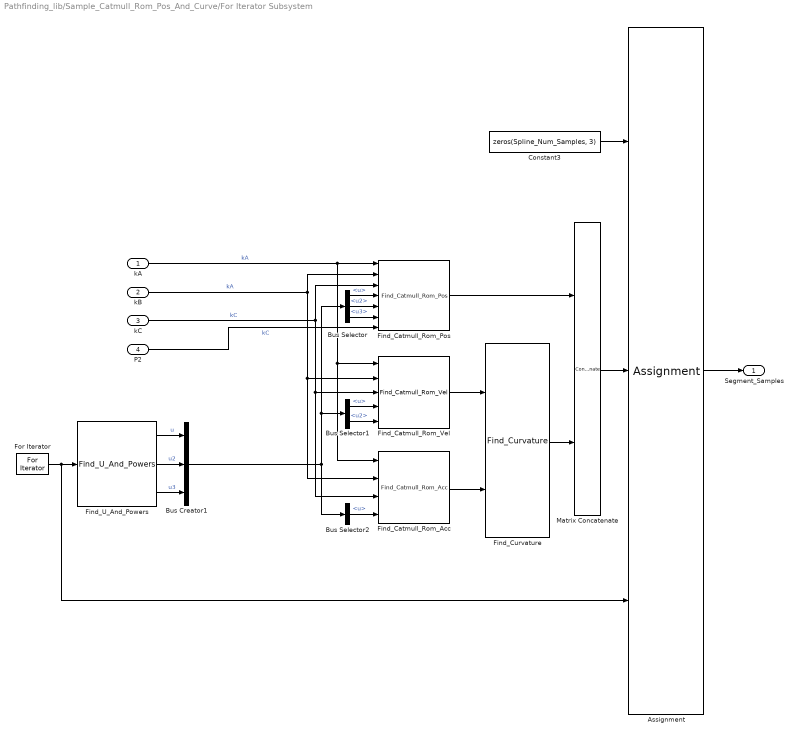
== system Pathfinding_lib/Sample_Catmull_Rom_Pos_And_Curve/For Iterator Subsystem ==
  kA : Inport  PortDimensions=[1 2]
  kB : Inport  Port=2  PortDimensions=[1 2]
  kC : Inport  Port=3  PortDimensions=[1 2]
  P2 : Inport  Port=4  PortDimensions=[1 2]
  Assignment : Assignment  NumberOfDimensions=2  DiagnosticForDimensions=Warning  IndexOptions=Index vector (port),Assign all  Indices=1,1  OutputSizes=1,1
  Bus Creator1 : BusCreator  Inputs=3
  Bus Selector : BusSelector  OutputSignals=u,u2,u3
  Bus Selector1 : BusSelector  OutputSignals=u,u2
  Bus Selector2 : BusSelector  OutputSignals=u
  Constant3 : Constant  Value=zeros(Spline_Num_Samples, 3)
  Find_Catmull_Rom_Acc : $bdroot/Find_Catmull_Rom_Acc  SystemSampleTime=-1  VariantActivationTime=update diagram  AllowFlexibleInterface=on  Latency=0  AutoFrameSizeCalculation=off
  Find_Catmull_Rom_Pos : $bdroot/Find_Catmull_Rom_Pos  SystemSampleTime=-1  VariantActivationTime=update diagram  AllowFlexibleInterface=on  Latency=0  AutoFrameSizeCalculation=off
  Find_Catmull_Rom_Vel : $bdroot/Find_Catmull_Rom_Vel  SystemSampleTime=-1  VariantActivationTime=update diagram  AllowFlexibleInterface=on  Latency=0  AutoFrameSizeCalculation=off
  Find_Curvature : $bdroot/Find_Curvature  SystemSampleTime=-1  VariantActivationTime=update diagram  AllowFlexibleInterface=on  Latency=0  AutoFrameSizeCalculation=off
  Find_U_And_Powers : $bdroot/Find_U_And_Powers  SystemSampleTime=-1  VariantActivationTime=update diagram  AllowFlexibleInterface=on  Latency=0  AutoFrameSizeCalculation=off
  For Iterator : ForIterator  IterationLimit=Spline_Num_Samples
  Matrix Concatenate : Concatenate  Mode=Multidimensional array  ConcatenateDimension=2
  Segment_Samples : Outport
  wires:
  Find_U_And_Powers/3 -> Bus Creator1/3  "u3"
  Find_U_And_Powers/1 -> Bus Creator1/1  "u"
  Find_U_And_Powers/2 -> Bus Creator1/2  "u2"
  P2/1 -> Find_Catmull_Rom_Pos/7  "kC"
  Matrix Concatenate/1 -> Assignment/2
  Find_Catmull_Rom_Pos/1 -> Matrix Concatenate/1
  Find_Catmull_Rom_Acc/1 -> Find_Curvature/2
  Find_Catmull_Rom_Vel/1 -> Find_Curvature/1
  kC/1 -> Find_Catmull_Rom_Vel/3, Find_Catmull_Rom_Acc/3, Find_Catmull_Rom_Pos/3  "kC"
  kB/1 -> Find_Catmull_Rom_Pos/2, Find_Catmull_Rom_Acc/2, Find_Catmull_Rom_Vel/2  "kA"
  kA/1 -> Find_Catmull_Rom_Pos/1, Find_Catmull_Rom_Vel/1, Find_Catmull_Rom_Acc/1  "kA"
  Bus Selector2/1 -> Find_Catmull_Rom_Acc/4  "<u>"
  Bus Selector1/2 -> Find_Catmull_Rom_Vel/5  "<u2>"
  Bus Selector1/1 -> Find_Catmull_Rom_Vel/4  "<u>"
  Bus Selector/2 -> Find_Catmull_Rom_Pos/5  "<u2>"
  Bus Selector/3 -> Find_Catmull_Rom_Pos/6  "<u3>"
  Bus Selector/1 -> Find_Catmull_Rom_Pos/4  "<u>"
  Bus Creator1/1 -> Bus Selector2/1, Bus Selector1/1, Bus Selector/1
  Assignment/1 -> Segment_Samples/1
  Constant3/1 -> Assignment/1
  For Iterator/1 -> Assignment/3, Find_U_And_Powers/1
  Find_Curvature/1 -> Matrix Concatenate/2
  ? -> ?

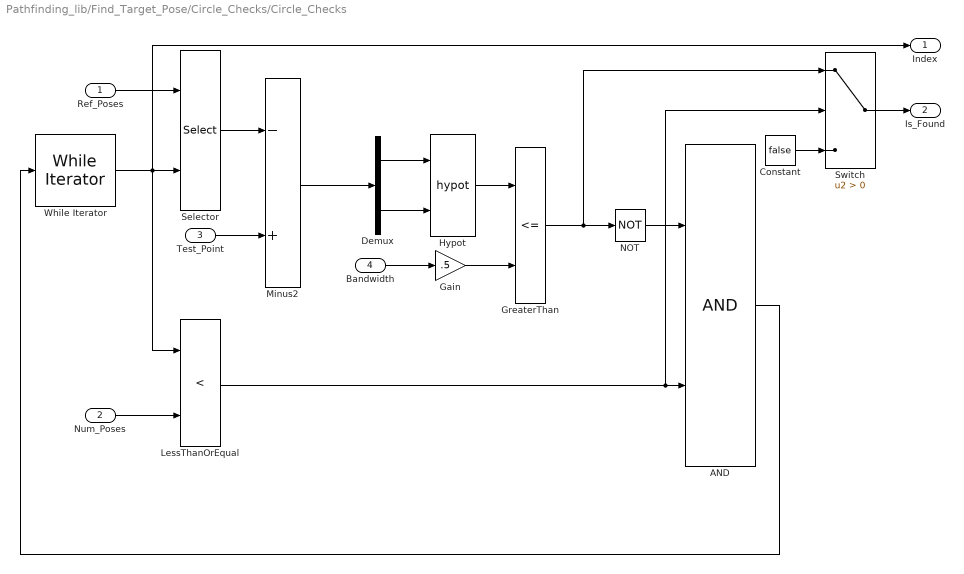
== system Pathfinding_lib/Find_Target_Pose/Circle_Checks/Circle_Checks ==
  Ref_Poses : Inport
  Num_Poses : Inport  Port=2
  Test_Point : Inport  Port=3
  Bandwidth : Inport  Port=4
  AND : Logic  IconShape=distinctive  AllPortsSameDT=off  OutDataTypeStr=boolean
  Constant : Constant  Value=false
  Demux : Demux  Outputs=2
  Gain : Gain  Gain=.5
  GreaterThan : RelationalOperator  Operator=<=  OutDataTypeStr=boolean  RndMeth=Simplest  InputSameDT=off
  Hypot : Math  Operator=hypot
  LessThanOrEqual : RelationalOperator  Operator=<  OutDataTypeStr=boolean  RndMeth=Simplest  InputSameDT=off
  Minus2 : Sum  Inputs=-+
  NOT : Logic  Operator=NOT  IconShape=distinctive  AllPortsSameDT=off  OutDataTypeStr=boolean
  Selector : Selector  NumberOfDimensions=2  InputPortWidth=3  IndexOptions=Index vector (port),Select all  Indices=[1 3],1  OutputSizes=1,1
  Switch : Switch  Criteria=u2 > Threshold  SaturateOnIntegerOverflow=off  InputSameDT=off
  While Iterator : WhileIterator  MaxIters=Spline_Max_Num_RefPoses  WhileBlockType=do-while  ShowIterationPort=on
  Index : Outport
  Is_Found : Outport  Port=2
  wires:
  Demux/1 -> Hypot/1
  Num_Poses/1 -> LessThanOrEqual/2
  LessThanOrEqual/1 -> Switch/2, AND/2
  Selector/1 -> Minus2/1
  Ref_Poses/1 -> Selector/1
  Test_Point/1 -> Minus2/2
  Minus2/1 -> Demux/1
  Demux/2 -> Hypot/2
  Bandwidth/1 -> Gain/1
  Hypot/1 -> GreaterThan/1
  Gain/1 -> GreaterThan/2
  GreaterThan/1 -> Switch/1, NOT/1
  AND/1 -> While Iterator/1
  While Iterator/1 -> LessThanOrEqual/1, Selector/2, Index/1
  NOT/1 -> AND/1
  Switch/1 -> Is_Found/1
  Constant/1 -> Switch/3

== matlab function Pathfinding_lib/Find_Curvature/MATLAB Function ==
  data: u input size=[2 2]; y output size=1
function y = Determinant(u)

y = u(1,1)*u(2,2)-u(2,1)*u(1,2);
